simulink model "Stepper_Model_2017_mark"  (R2017a)
settings: Solver=VariableStepAuto  StartTime=0.0  StopTime=tsim  RelTol=1e-3
model workspace (MAT data in the model file):
  V = Simulink.Signal
  V.DataType = 'auto'
  V.Dimensions = -1
  V.DimensionsMode = 'auto'
  V.Complexity = 'auto'
  V.SampleTime = -1
  V.SamplingMode = 'auto'
values from neighbouring files (symbols this model uses):
  c = 0.05    [K_Gain_matrix.m]    (also in Stepper_Model_2017_10_31_Script.m = 0.017; Stepper_Model_2017_Mark_Script.m)
  g = 9.82    [Stepper_Model_2017_10_31_Script.m]    (also in Stepper_Model_2017_Mark_Script.m)
  K = place(A,B,poles)    [K_Gain_matrix.m]    (also in Stepper_Model_2017_10_31_Script.m; Stepper_Model_2017_Mark_Script.m)
  L = 0.8    [K_Gain_matrix.m]    (also in Stepper_Model_2017_10_31_Script.m = 1.06; Stepper_Model_2017_Mark_Script.m)
  m = 0.2    [K_Gain_matrix.m]    (also in Stepper_Model_2017_10_31_Script.m; Stepper_Model_2017_Mark_Script.m)
  N = N(4:end)    [Lab2.m]    (also in Stepper_Model_2017_10_31_Script.m = 1/((C-D*K)/(B*K-A)*B+D); Stepper_Model_2017_Mark_Script.m = 1/((C-D*K)/(B*K-A)*B+D))
  theta0 = startAngle*pi/180    (= 0.0872664625997)    [Stepper_Model_2017_10_31_Script.m]    (also in Stepper_Model_2017_Mark_Script.m)
undefined symbols (not defined in the file or in its folder): sigbuilder_block
settings Model: Creator=Administrator  LastModifiedBy=Mark

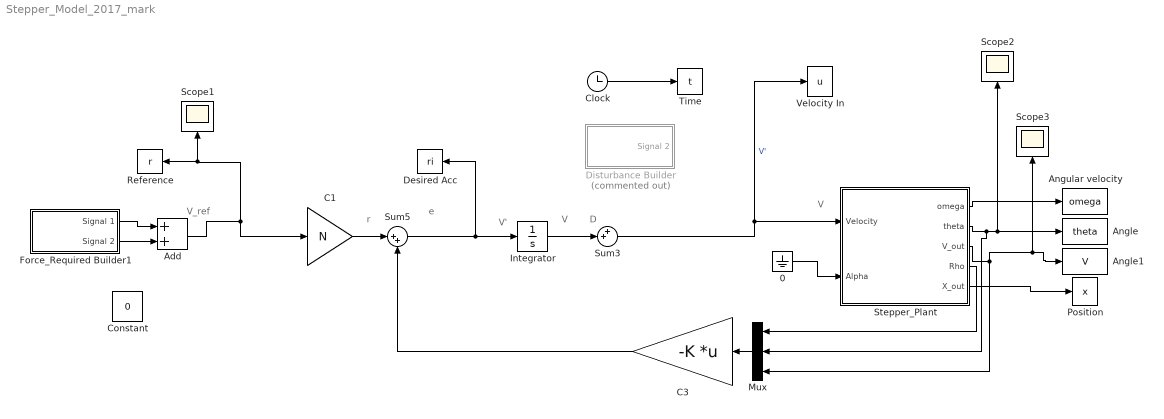
== system Stepper_Model_2017_mark ==
  note: V
  note: V'
  note: V
  note: V_ref
  note: D
  note: e
  note: r
  0 : Ground
  Add : Sum
  Angle : ToWorkspace  VariableName=theta  SampleTime=-1
  Angle1 : ToWorkspace  VariableName=V  SampleTime=-1
  Angular velocity : ToWorkspace  VariableName=omega  SampleTime=-1
  C1 : Gain  Gain=N
  C3 : Gain  Gain=-K  Multiplication=Matrix(K*u) (u vector)
  Clock : Clock
  Constant : Constant  Value=0
  Desired Acc : ToWorkspace  VariableName=ri  SampleTime=-1
  Disturbance Builder : Subsystem  Tag=STV Subsys  Commented=on  LoadFcn=sigbuilder_block('load');  StartFcn=sigbuilder_block('start');  StopFcn=sigbuilder_block('stop');  ClipboardFcn=sigbuilder_block('clipboard');  mask(Sigbuilder block){tuvar=[0:10]}
      mask help: Simulink:masks:SigbuilderBlock_MD
      mask init:
      | if ~strcmp(get_param(bdroot(gcbh),'SimulationStatus'),'stopped') tuvar = sigbuilder_block('maskInit'); end
      settings: CopyFcn=sigbuilder_block('copy');  DeleteFcn=sigbuilder_block('delete');  ModelCloseFcn=sigbuilder_block('modelClose');  PreSaveFcn=sigbuilder_block('preSave');  PauseFcn=sigbuilder_block('pause');  ContinueFcn=sigbuilder_block('continue');  NameChangeFcn=sigbuilder_block('namechange');  OpenFcn=sigbuilder_block('open',[203 87.5 550.5 362.5 ]);  CloseFcn=sigbuilder_block('close');
      mask Display: plot(0, 0, 100, 100,[2, 2, 32, 32, 2], [68, 8, 8, 68, 68],[32, 2], [38, 38], [32, 19, 2],[53, 60, 44], [32, 17, 17, 2],[16, 16, 31, 31]);txt = getActiveGroup(gcbh);text(2, 100, txt,'verticalAlignment', 'top');
  Force_Required Builder1 : Subsystem  Tag=STV Subsys  LoadFcn=sigbuilder_block('load');  StartFcn=sigbuilder_block('start');  StopFcn=sigbuilder_block('stop');  ClipboardFcn=sigbuilder_block('clipboard');  mask(Sigbuilder block){tuvar=[0:10]}
      mask help: Simulink:masks:SigbuilderBlock_MD
      mask init:
      | if ~strcmp(get_param(bdroot(gcbh),'SimulationStatus'),'stopped') tuvar = sigbuilder_block('maskInit'); end
      settings: CopyFcn=sigbuilder_block('copy');  DeleteFcn=sigbuilder_block('delete');  ModelCloseFcn=sigbuilder_block('modelClose');  PreSaveFcn=sigbuilder_block('preSave');  PauseFcn=sigbuilder_block('pause');  ContinueFcn=sigbuilder_block('continue');  NameChangeFcn=sigbuilder_block('namechange');  OpenFcn=sigbuilder_block('open',[520.5 84.75 550.5 362.25 ]);  CloseFcn=sigbuilder_block('close');
      mask Display: plot(0, 0, 100, 100,[2, 2, 32, 32, 2], [68, 8, 8, 68, 68],[32, 2], [38, 38], [32, 19, 2],[53, 60, 44], [32, 17, 17, 2],[16, 16, 31, 31]);txt = getActiveGroup(gcbh);text(2, 100, txt,'verticalAlignment', 'top');
  Integrator : Integrator  InitialCondition=0.01
  Mux : Mux  Inputs=3
  Position : ToWorkspace  VariableName=x  SampleTime=-1
  Reference : ToWorkspace  VariableName=r  SampleTime=-1
  Scope1 : Scope
  Scope2 : Scope
  Scope3 : Scope
  Stepper_Plant : Subsystem
  Sum3 : Sum  Inputs=++|
  Sum5 : Sum  Inputs=|++
  Time : ToWorkspace  VariableName=t  SampleTime=-1
  Velocity In : ToWorkspace  VariableName=u  SampleTime=-1
  wires:
  0/1 -> Stepper_Plant/2(Alpha)
  Clock/1 -> Time/1
  Stepper_Plant/1(omega) -> Angular velocity/1
  Stepper_Plant/5(X_out) -> Position/1
  Stepper_Plant/2(theta) -> Mux/2, Scope2/1, Angle/1
  C3/1 -> Sum5/2
  Sum3/1 -> Velocity In/1, Stepper_Plant/1(Velocity)  "V'"
  Add/1 -> C1/1, Scope1/1, Reference/1
  C1/1 -> Sum5/1
  Force_Required Builder1/1(Signal 1) -> Add/1
  Force_Required Builder1/2(Signal 2) -> Add/2
  Stepper_Plant/3(V_out) -> Mux/3, Scope3/1, Angle1/1
  Sum5/1 -> Desired Acc/1, Integrator/1
  Integrator/1 -> Sum3/2
  Mux/1 -> C3/1
  Stepper_Plant/4(Rho) -> Mux/1

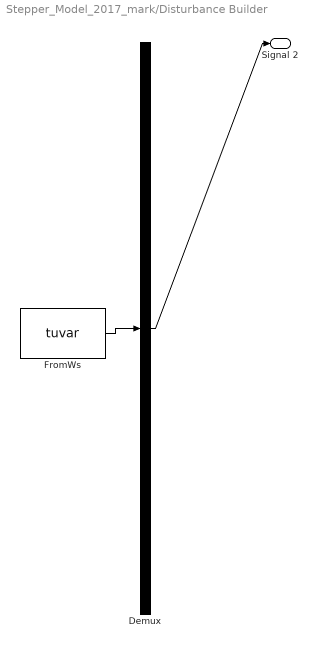
== system Stepper_Model_2017_mark/Disturbance Builder ==
  Demux : Demux  Tag=STV Demux  Outputs=1
  FromWs : FromWorkspace  Tag=STV FromWs  VariableName=tuvar  SampleTime=0
      SigBuilderData=|
      | common.afterFinalStr = 'Extrapolate'
      | common.sampleTime = 0
      | dataSet.timeRange = [0 10]
      | dataSet.name = 'Group 1'
      | sbobj.Groups.Name = 'Group 1'
      | sbobj.Groups.Signals.Name = 'Signal 2'
      | sbobj.Groups.Signals.XData = [0 10]
      | sbobj.Groups.Signals.YData = [0 0]
  Signal 2 : Outport  Tag=STV Outport
  wires:
  FromWs/1 -> Demux/1
  Demux/1 -> Signal 2/1

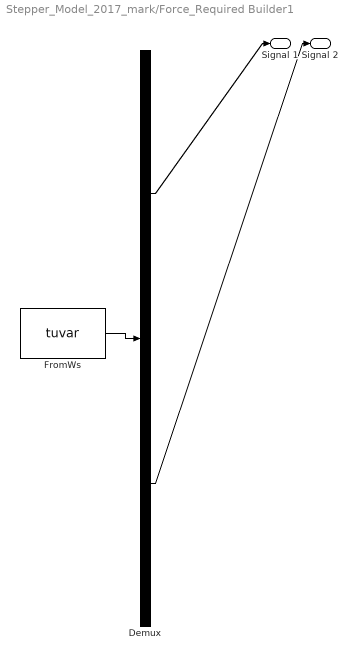
== system Stepper_Model_2017_mark/Force_Required Builder1 ==
  Demux : Demux  Tag=STV Demux  Outputs=2
  FromWs : FromWorkspace  Tag=STV FromWs  VariableName=tuvar  SampleTime=0
      SigBuilderData=|
      | common.afterFinalStr = 'Extrapolate'
      | common.sampleTime = 0
      | dataSet.timeRange = [0 10]
      | dataSet.name = 'Group 1'
      | sbobj.Groups.Name = 'Group 1'
      | sbobj.Groups.Signals(1).Name = 'Signal 1'
      | sbobj.Groups.Signals(1).XData = [0 10]
      | sbobj.Groups.Signals(1).YData = [0 0]
      | sbobj.Groups.Signals(2).Name = 'Signal 2'
      | sbobj.Groups.Signals(2).XData = [0 4 4 6 6 10]
      | sbobj.Groups.Signals(2).YData = [0 0 0.44 0.44 0 0]
  Signal 1 : Outport  Tag=STV Outport
  Signal 2 : Outport  Tag=STV Outport  Port=2
  wires:
  FromWs/1 -> Demux/1
  Demux/1 -> Signal 1/1
  Demux/2 -> Signal 2/1

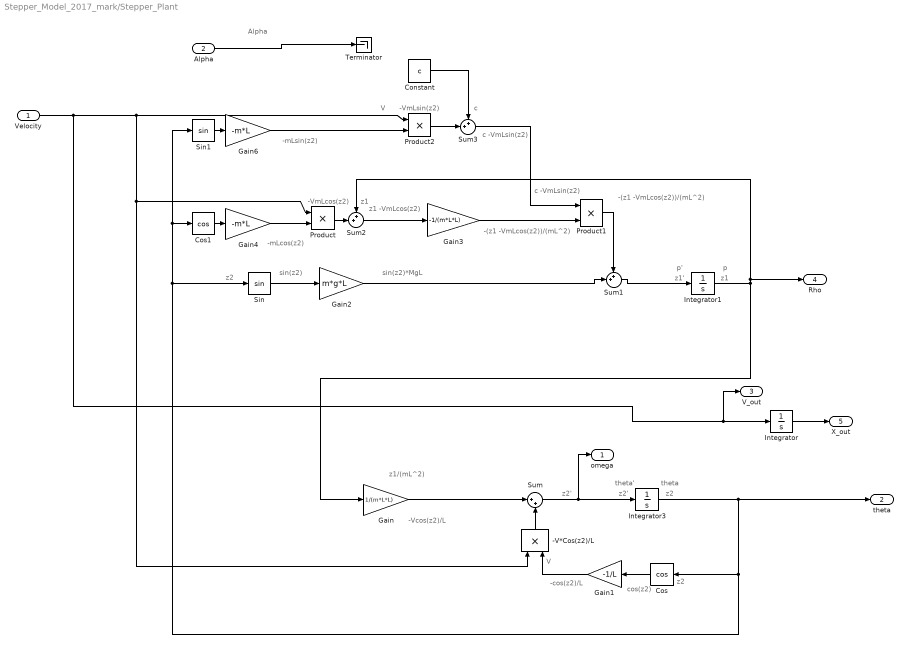
== system Stepper_Model_2017_mark/Stepper_Plant ==
  note: -mLcos(z2)
  note: V
  note: z1 -VmLcos(z2)
  note: sin(z2)*MgL
  note: sin(z2)
  note: -VmLcos(z2)
  note: z1
  note: z2'
  note: z1/(mL^2)
  note: -Vcos(z2)/L
  note: -cos(z2)/L
  note: cos(z2)
  note: z2
  note: V
  note: z2
  note: z2'
  note: z1
  note: z1'
  note: theta
  note: p
  note: theta'
  note: p'
  note: z2
  note: Alpha
  note: -(z1 -VmLcos(z2))/(mL^2)
  note: c
  note: -mLsin(z2)
  note: -VmLsin(z2)
  note: c -VmLsin(z2)
  note: c -VmLsin(z2)
  note: -(z1 -VmLcos(z2))/(mL^2)
  Velocity : Inport
  Alpha : Inport  Port=2
  -V*Cos(z2)/L : Product
  Constant : Constant  Value=c
  Cos : Trigonometry  Operator=cos
  Cos1 : Trigonometry  Operator=cos
  Gain : Gain  Gain=1/(m*L*L)
  Gain1 : Gain  Gain=-1/L
  Gain2 : Gain  Gain=m*g*L
  Gain3 : Gain  Gain=-1/(m*L*L)
  Gain4 : Gain  Gain=-m*L
  Gain6 : Gain  Gain=-m*L
  Integrator : Integrator
  Integrator1 : Integrator
  Integrator3 : Integrator  InitialCondition=theta0
  Product : Product
  Product1 : Product
  Product2 : Product
  Sin : Trigonometry
  Sin1 : Trigonometry
  Sum : Sum  Inputs=|++
  Sum1 : Sum  Inputs=++|
  Sum2 : Sum  Inputs=++|
  Sum3 : Sum  Inputs=++|
  Terminator : Terminator
  omega : Outport
  theta : Outport  Port=2
  V_out : Outport  Port=3
  Rho : Outport  Port=4
  X_out : Outport  Port=5
  wires:
  Sum1/1 -> Integrator1/1
  Gain4/1 -> Product/2
  Cos/1 -> Gain1/1
  Sin/1 -> Gain2/1
  Sum2/1 -> Gain3/1
  Gain3/1 -> Product1/2
  Gain2/1 -> Sum1/2
  Product/1 -> Sum2/2
  Integrator1/1 -> Rho/1, Sum2/1, Gain/1
  Integrator3/1 -> Cos/1, Sin/1, Cos1/1, Sin1/1, theta/1
  Sum/1 -> omega/1, Integrator3/1
  Gain/1 -> Sum/1
  Alpha/1 -> Terminator/1
  Velocity/1 -> Integrator/1, V_out/1, Product/1, -V*Cos(z2)/L/1, Product2/1
  Gain1/1 -> -V*Cos(z2)/L/2
  -V*Cos(z2)/L/1 -> Sum/2
  Sum3/1 -> Product1/1
  Product2/1 -> Sum3/2
  Gain6/1 -> Product2/2
  Cos1/1 -> Gain4/1
  Sin1/1 -> Gain6/1
  Constant/1 -> Sum3/1
  Product1/1 -> Sum1/1
  Integrator/1 -> X_out/1
